simulink model "onelink_simscape"  (R2025a)
settings: Solver=ode15s  StartTime=0.0  StopTime=10  RelTol=1e-4
libraries: fl_lib x179, ee_lib x62, nesl_utility x15
(part 1 of 2)
settings Model: Creator=yang  LastModifiedBy=yang

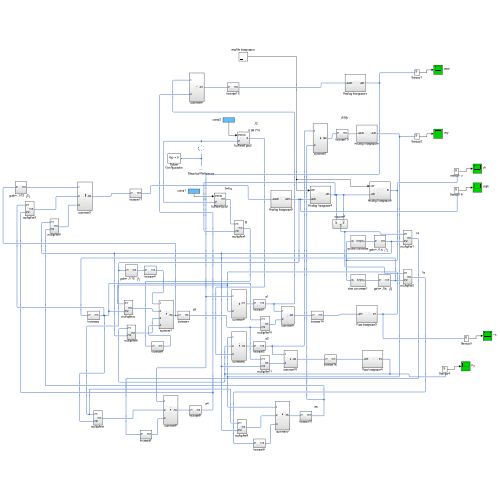
[thumbnail: Simulink's stored preview of the top-level diagram]
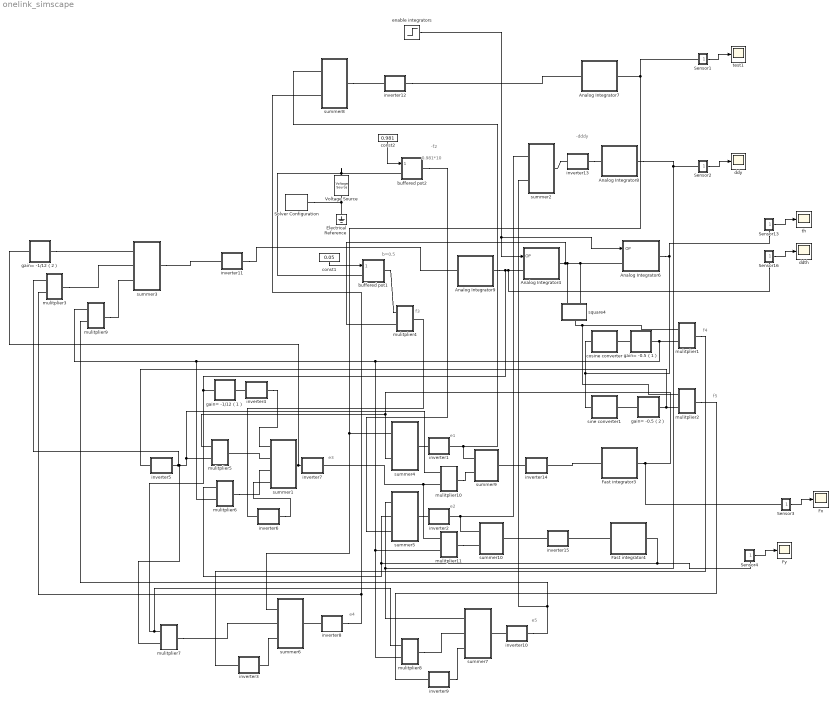
== system onelink_simscape ==
  note: 0.981*10
  note: -dddy
  note: e5
  note: e4
  note: e1
  note: f4
  note: f3
  note: b=0.5
  note: -f2
  note: f5
  note: e2
  note: e3
  Analog Integrator4 : Subsystem
  Analog Integrator6 : Subsystem
  Analog Integrator7 : Subsystem
  Analog Integrator8 : Subsystem
  Analog Integrator9 : Subsystem
  Electrical Reference : fl_lib/Electrical/Electrical Elements/Electrical Reference
  Fast integrator3 : Subsystem
  Fast integrator4 : Subsystem
  Fx : Scope
      settings: ActiveDisplayYMinimum=-37.571328229852568  ActiveDisplayYMaximum=27.796484303991519  DataLoggingVariableName=ScopeData4
  Fy : Scope
      settings: ActiveDisplayYMinimum=-21.350757214154832  ActiveDisplayYMaximum=2.3911956510501242  DataLoggingVariableName=ScopeData5
  Sensor1 : Subsystem
      mask Display: disp('S')
  Sensor13 : Subsystem
      settings: PortSchema="{\"entries\":[{\"content\":{\"sides\":[{\"content\":{},\"type\":\"ConnectorPlacement.EquallySpacedRectSide\",\"uuid\":\"8056b96b-3671-4774-a535-635e6b55e7ce\"},{\"content\":{\"connectorIds\":[\"Out1\"],\"side\":\"RIGHT\"},\"type\":\"ConnectorPlacement.EquallySpacedRectSide\",\"uuid\":\"d8cfde34-d3f1-4c6d-ab3a-246c7ad79664\"},{\"content\":{\"side\":\"TOP\"},\"type\":\"ConnectorPlacement.EquallySpacedRectSide\",\"uuid\":\"c78cfa8c-6b6c-49de-bc78-645cca7ac0e7\"},{\"content\":{\"connectorIds\":[\"RConn1\"],\"side\":\"BOTTOM\"},\"type\":\"ConnectorPlacement.EquallySpacedRectSide\",\"uuid\":\"959be980-bdc1-4803-beb2-1cc3f6e5a73d\"}]},\"type\":\"ConnectorPlacement.EquallySpacedConnector\",\"uuid\":\"4ae0772a-f601-42fd-b251-b1e340c12b80\"}],\"packageUris\":[\"http://schema.mathworks.com/mf0/Connector/R2020b\"],\"version\":\"1.0\"}"
      mask Display: disp('S')
  Sensor16 : Subsystem
      settings: PortSchema="{\"entries\":[{\"content\":{\"sides\":[{\"content\":{},\"type\":\"ConnectorPlacement.EquallySpacedRectSide\",\"uuid\":\"8056b96b-3671-4774-a535-635e6b55e7ce\"},{\"content\":{\"connectorIds\":[\"Out1\"],\"side\":\"RIGHT\"},\"type\":\"ConnectorPlacement.EquallySpacedRectSide\",\"uuid\":\"d8cfde34-d3f1-4c6d-ab3a-246c7ad79664\"},{\"content\":{\"side\":\"TOP\"},\"type\":\"ConnectorPlacement.EquallySpacedRectSide\",\"uuid\":\"c78cfa8c-6b6c-49de-bc78-645cca7ac0e7\"},{\"content\":{\"connectorIds\":[\"RConn1\"],\"side\":\"BOTTOM\"},\"type\":\"ConnectorPlacement.EquallySpacedRectSide\",\"uuid\":\"959be980-bdc1-4803-beb2-1cc3f6e5a73d\"}]},\"type\":\"ConnectorPlacement.EquallySpacedConnector\",\"uuid\":\"4ae0772a-f601-42fd-b251-b1e340c12b80\"}],\"packageUris\":[\"http://schema.mathworks.com/mf0/Connector/R2020b\"],\"version\":\"1.0\"}"
      mask Display: disp('S')
  Sensor2 : Subsystem
      mask Display: disp('S')
  Sensor3 : Subsystem
      mask Display: disp('S')
  Sensor4 : Subsystem
      settings: PortSchema="{\"entries\":[{\"content\":{\"sides\":[{\"content\":{},\"type\":\"ConnectorPlacement.EquallySpacedRectSide\",\"uuid\":\"8056b96b-3671-4774-a535-635e6b55e7ce\"},{\"content\":{\"connectorIds\":[\"Out1\"],\"side\":\"RIGHT\"},\"type\":\"ConnectorPlacement.EquallySpacedRectSide\",\"uuid\":\"d8cfde34-d3f1-4c6d-ab3a-246c7ad79664\"},{\"content\":{\"side\":\"TOP\"},\"type\":\"ConnectorPlacement.EquallySpacedRectSide\",\"uuid\":\"c78cfa8c-6b6c-49de-bc78-645cca7ac0e7\"},{\"content\":{\"connectorIds\":[\"RConn1\"],\"side\":\"BOTTOM\"},\"type\":\"ConnectorPlacement.EquallySpacedRectSide\",\"uuid\":\"959be980-bdc1-4803-beb2-1cc3f6e5a73d\"}]},\"type\":\"ConnectorPlacement.EquallySpacedConnector\",\"uuid\":\"4ae0772a-f601-42fd-b251-b1e340c12b80\"}],\"packageUris\":[\"http://schema.mathworks.com/mf0/Connector/R2020b\"],\"version\":\"1.0\"}"
      mask Display: disp('S')
  Solver Configuration : nesl_utility/Solver Configuration  PhysicalDomain=network_engine_domain  SubClassName=solver  LeftPortType=input  RightPortType=generic  Tones=[]  Harmonics=[]  SimulateNoise=off  Profile=off  UseLocalSampling=off  EnableSwitchedLinearOptims=on  FrequencyDomain=off  UseCCode=off  RelTol=0.001  AbsTol=1e-06  MinStep=1e-09  ToWorkspace=off  RevertToSquareIcSolve=off  NumHomotopyIterations=100  PhasorMode=off  PhasorModeNumHarmonics=1  ConsistencySolver=NEWTON_XTOL_AFTER_FTOL  IndexReductionMethod=DerivativeReplacement  DoDC=off  ResidualTolerance=1e-09  ConsistencyTolSource=GLOBAL  ConsistencyAbsTol=0.001  ConsistencyRelTol=0.001  ConsistencyTolFactor=0.001  UseLocalSolver=off  LocalSolverChoice=NE_BACKWARD_EULER_ADVANCER  ResolveIndetEquations=on  FunctionEvalNumThread=1  LocalSolverSampleTime=0.001  DoFixedCost=off  MaxNonlinIter=3  MaxModeIter=2  ComputeImpulses=off  ImpulseIterations=2  LinearAlgebra=auto  LinearAlgebraNumThread=0  EquationFormulation=NE_TIME_EF  DelaysMemoryBudget=1024  AutomaticFiltering=on  FilteringTimeConstant=0.001  PartitionStorageMethod=AS_NEEDED  PartitionMemoryBudget=1024  PartitionMethod=ROBUST  MultibodyUseLocalSolver=off  MultibodyLocalSolverChoice=ODE1  MultibodyLocalSolverSampleTime=0.001
  Voltage Source : ee_lib/Sources/Voltage Source  dc_voltage=10 V  ac_voltage=0 V  ac_shift=0 rad  ac_frequency=60 Hz  noise_mode=ee.enum.sources.noise.Disabled  PSD=0 V^2/Hz  sample_time=1e-3 s  repeatability=ee.enum.sources.repeatability.NotRepeatable  user_seed=0  auto_seed=3499211588  i_specify=off  i_priority=None  i=0 A  i_nominal_specify=off  i_nominal_value=1  i_nominal_unit=A  v_specify=off  v_priority=None  v=0 V  v_nominal_specify=off  v_nominal_value=1  v_nominal_unit=V
  buffered pot1 : Subsystem
  buffered pot2 : Subsystem
  const1 : Constant  Value=0.05
  const2 : Constant  Value=0.981
  cosine converter : Subsystem
  ddth : Scope
      settings: ActiveDisplayYMinimum=-17.651400313660709  ActiveDisplayYMaximum=14.639431018318287
  ddy : Scope
      settings: ActiveDisplayYMinimum=-8.0449324202485482  ActiveDisplayYMaximum=0.91267312902724274  DataLoggingVariableName=ScopeData3
  enable integrators : Step  Time=0.02  SampleTime=0
  gain= -0.5（1） : Subsystem
  gain= -0.5（2） : Subsystem
  gain= -1/12（1） : Subsystem
  gain= -1/12（2） : Subsystem
  inverter1 : Subsystem
  inverter10 : Subsystem
  inverter11 : Subsystem
  inverter12 : Subsystem
  inverter13 : Subsystem
  inverter14 : Subsystem
  inverter15 : Subsystem
  inverter2 : Subsystem
  inverter3 : Subsystem
  inverter4 : Subsystem
  inverter5 : Subsystem
  inverter6 : Subsystem
  inverter7 : Subsystem
  inverter8 : Subsystem
  inverter9 : Subsystem
  mulitplier1 : Subsystem
  mulitplier10 : Subsystem
  mulitplier11 : Subsystem
  mulitplier2 : Subsystem
  mulitplier3 : Subsystem
  mulitplier4 : Subsystem
  mulitplier5 : Subsystem
  mulitplier6 : Subsystem
  mulitplier7 : Subsystem
  mulitplier8 : Subsystem
  mulitplier9 : Subsystem
  sine converter1 : Subsystem
  square4 : Subsystem
  summer1 : Subsystem
  summer10 : Subsystem
  summer2 : Subsystem
  summer3 : Subsystem
  summer4 : Subsystem
  summer5 : Subsystem
  summer6 : Subsystem
  summer7 : Subsystem
  summer8 : Subsystem
  summer9 : Subsystem
  test1 : Scope
      settings: ActiveDisplayYMinimum=-5.82803  ActiveDisplayYMaximum=0.09194
  th : Scope
      settings: ActiveDisplayYMinimum=-2.64598748843829  ActiveDisplayYMaximum=0.29399860983456916  DataLoggingVariableName=ScopeData14
  wires:
  const2/1 -> buffered pot2/1(input0)
  enable integrators/1 -> Analog Integrator6/1(OP), Analog Integrator4/1(OP)
  const1/1 -> buffered pot1/1(input0)
  Sensor16/1(Out1) -> ddth/1
  Sensor1/1(Out1) -> test1/1
  Sensor2/1(Out1) -> ddy/1
  Sensor3/1(Out1) -> Fx/1
  Sensor4/1(Out1) -> Fy/1
  Sensor13/1(Out1) -> th/1
  connections:
  Solver Configuration/RConn1 -- Voltage Source/RConn1 -- Electrical Reference/LConn1
  Voltage Source/LConn1 -- buffered pot1/LConn1 -- buffered pot2/LConn1
  Analog Integrator4/RConn1 -- mulitplier4/LConn2 -- square4/LConn1 -- square4/LConn2 -- Analog Integrator6/LConn1
  buffered pot1/RConn1 -- mulitplier4/LConn1
  mulitplier1/LConn1 -- mulitplier2/LConn1 -- square4/RConn1
  Analog Integrator6/RConn1 -- sine converter1/LConn1 -- cosine converter/LConn1 -- Sensor13/RConn1
  Analog Integrator9/RConn1 -- Sensor16/RConn1 -- Analog Integrator4/LConn1 -- mulitplier8/LConn1 -- mulitplier7/LConn1 -- gain= -1/12（1）/LConn1
  summer4/LConn1 -- summer6/LConn1 -- Sensor1/LConn1 -- Analog Integrator7/RConn1
  Fast integrator3/RConn1 -- Sensor3/LConn1 -- mulitplier5/LConn1 -- summer4/LConn2
  inverter1/LConn1 -- summer4/RConn1
  Analog Integrator8/RConn1 -- Sensor2/LConn1 -- summer7/LConn1 -- summer5/LConn1
  summer5/LConn2 -- mulitplier6/LConn1 -- Sensor4/RConn1 -- Fast integrator4/RConn1
  buffered pot2/RConn1 -- summer5/LConn3
  inverter2/LConn1 -- summer5/RConn1
  inverter4/LConn1 -- gain= -1/12（1）/RConn1
  inverter4/RConn1 -- summer1/LConn1
  gain= -0.5（1）/LConn1 -- cosine converter/RConn1
  mulitplier1/LConn2 -- mulitplier11/LConn2 -- mulitplier8/LConn2 -- mulitplier9/LConn1 -- mulitplier6/LConn2 -- gain= -0.5（1）/RConn1
  gain= -0.5（2）/LConn1 -- sine converter1/RConn1
  mulitplier2/LConn2 -- inverter5/LConn1 -- gain= -0.5（2）/RConn1
  inverter5/RConn1 -- mulitplier3/LConn1 -- mulitplier7/LConn2 -- mulitplier10/LConn1 -- mulitplier5/LConn2
  summer1/LConn2 -- mulitplier5/RConn1
  mulitplier6/RConn1 -- summer1/LConn3
  inverter6/LConn1 -- mulitplier4/RConn1
  inverter6/RConn1 -- summer1/LConn4
  inverter7/LConn1 -- gain= -1/12（2）/LConn1 -- summer1/RConn1
  mulitplier7/RConn1 -- summer6/LConn2
  mulitplier1/RConn1 -- inverter3/LConn1
  summer6/LConn3 -- inverter3/RConn1
  inverter8/LConn1 -- summer6/RConn1
  mulitplier8/RConn1 -- summer7/LConn2
  mulitplier2/RConn1 -- inverter9/LConn1
  inverter9/RConn1 -- summer7/LConn3
  inverter10/LConn1 -- summer7/RConn1
  summer8/LConn1 -- summer9/LConn1 -- inverter1/RConn1
  inverter8/RConn1 -- mulitplier3/LConn2 -- summer8/LConn2
  summer8/RConn1 -- inverter12/LConn1
  inverter12/RConn1 -- Analog Integrator7/LConn1
  summer2/LConn1 -- summer10/LConn1 -- inverter2/RConn1
  inverter10/RConn1 -- mulitplier9/LConn2 -- summer2/LConn2
  inverter13/LConn1 -- summer2/RConn1
  inverter13/RConn1 -- Analog Integrator8/LConn1
  gain= -1/12（2）/RConn1 -- summer3/LConn1
  mulitplier3/RConn1 -- summer3/LConn2
  mulitplier9/RConn1 -- summer3/LConn3
  mulitplier10/LConn2 -- inverter7/RConn1 -- mulitplier11/LConn1
  mulitplier10/RConn1 -- summer9/LConn2
  inverter14/LConn1 -- summer9/RConn1
  Fast integrator3/LConn1 -- inverter14/RConn1
  inverter15/LConn1 -- summer10/RConn1
  Fast integrator4/LConn1 -- inverter15/RConn1
  mulitplier11/RConn1 -- summer10/LConn2
  summer3/RConn1 -- inverter11/LConn1
  inverter11/RConn1 -- Analog Integrator9/LConn1

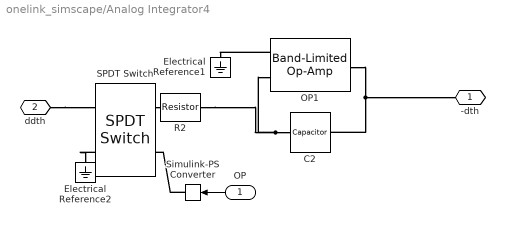
== system onelink_simscape/Analog Integrator4 ==
  OP : Inport
  C2 : ee_lib/Passive/Capacitor  cap_option=ee.enum.passive.capacitor.capOption.const  c=1e-6 F  Cvec=[1e-05, 1e-06] F  Vvec=[0, 10] V  CV_table_symmetry=ee.enum.passive.capacitor.tableSymmetry.yes  f_vec=[1, 10] kHz  DFext_vec=[.8, 1.2]  enable_C_tol=ee.enum.toleranceApplication.none  averaging_period=0 s  C_tol=5  tol_distribution=ee.enum.toleranceDistribution.uniform  nSigma=4  r=1e-6 Ohm  g=0 1/Ohm  enable_operating_limits=ee.enum.enable.no  operating_limit_action=ee.enum.passive.reportOpLim.warn  max_working_voltage_range=[-25, 25] V  power_rating=1 W  maxTemperature=85 degC  thermalEnable=false  thermalMass=1 J/K  i_specify=off  i_priority=None  i=0 A  i_nominal_specify=off  i_nominal_value=1  i_nominal_unit=A  v_specify=off  v_priority=High  v=1 V  v_nominal_specify=off  v_nominal_value=1  v_nominal_unit=V  vc_specify=on  vc_priority=High  vc=0 V  vc_nominal_specify=off  vc_nominal_value=1  vc_nominal_unit=V  T_specify=off  T_priority=None  T=298.15 K  T_nominal_specify=off  T_nominal_value=1  T_nominal_unit=K
  Electrical Reference1 : fl_lib/Electrical/Electrical Elements/Electrical Reference
  Electrical Reference2 : fl_lib/Electrical/Electrical Elements/Electrical Reference
  OP1 : ee_lib/Integrated Circuits/Band-Limited Op-Amp  A=1.8E6  Rin=1 GOhm  Rout=70 Ohm  Vmin=-15 V  Vmax=15 V  Vdotmax=2.8E6 V/s  f=8E6 Hz  V0=0 V
  R2 : fl_lib/Electrical/Electrical Elements/Resistor  R=1E6 Ohm  i_specify=off  i_priority=None  i=0 A  i_nominal_specify=off  i_nominal_value=1  i_nominal_unit=A  v_specify=off  v_priority=None  v=0 V  v_nominal_specify=off  v_nominal_value=1  v_nominal_unit=V
  SPDT Switch : ee_lib/Switches & Breakers/SPDT Switch  R_closed=0.01 Ohm  G_open=1e-6 S  Threshold=0.5 V  Width=0 V  model_dynamics=0  t_on=1e-3 s  t_off=1e-3 s  initial_vT=0 V
  Simulink-PS Converter : nesl_utility/Simulink-PS Converter  PhysicalDomain=network_engine_domain  SubClassName=ps_input  LeftPortType=input  RightPortType=output  PseudoPeriodic=off  Frequencies=[]  NoiseDistribution=none  NoiseParameters=[]  Unit=1  AffineConversion=off  FilteringAndDerivatives=provide  SimscapeFilterOrder=1  InputFilterTimeConstant=0.001  UdotUserProvided=0
  -dth : PMIOPort  Side=Right
  ddth : PMIOPort  Port=2  Side=Left
  wires:
  OP/1 -> Simulink-PS Converter/1
  connections:
  Simulink-PS Converter/RConn1 -- SPDT Switch/LConn1
  SPDT Switch/RConn1 -- Electrical Reference2/LConn1
  ddth/RConn1 -- SPDT Switch/RConn2
  SPDT Switch/LConn2 -- R2/LConn1
  OP1/RConn1 -- -dth/RConn1 -- C2/RConn1
  C2/LConn1 -- OP1/LConn2 -- R2/RConn1
  OP1/LConn1 -- Electrical Reference1/LConn1

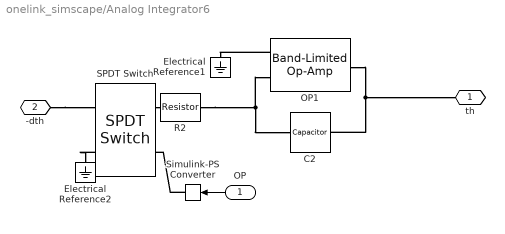
== system onelink_simscape/Analog Integrator6 ==
  OP : Inport
  C2 : ee_lib/Passive/Capacitor  cap_option=ee.enum.passive.capacitor.capOption.const  c=1e-6 F  Cvec=[1e-05, 1e-06] F  Vvec=[0, 10] V  CV_table_symmetry=ee.enum.passive.capacitor.tableSymmetry.yes  f_vec=[1, 10] kHz  DFext_vec=[.8, 1.2]  enable_C_tol=ee.enum.toleranceApplication.none  averaging_period=0 s  C_tol=5  tol_distribution=ee.enum.toleranceDistribution.uniform  nSigma=4  r=1e-6 Ohm  g=0 1/Ohm  enable_operating_limits=ee.enum.enable.no  operating_limit_action=ee.enum.passive.reportOpLim.warn  max_working_voltage_range=[-25, 25] V  power_rating=1 W  maxTemperature=85 degC  thermalEnable=false  thermalMass=1 J/K  i_specify=off  i_priority=None  i=0 A  i_nominal_specify=off  i_nominal_value=1  i_nominal_unit=A  v_specify=off  v_priority=High  v=1 V  v_nominal_specify=off  v_nominal_value=1  v_nominal_unit=V  vc_specify=on  vc_priority=High  vc=0 V  vc_nominal_specify=off  vc_nominal_value=1  vc_nominal_unit=V  T_specify=off  T_priority=None  T=298.15 K  T_nominal_specify=off  T_nominal_value=1  T_nominal_unit=K
  Electrical Reference1 : fl_lib/Electrical/Electrical Elements/Electrical Reference
  Electrical Reference2 : fl_lib/Electrical/Electrical Elements/Electrical Reference
  OP1 : ee_lib/Integrated Circuits/Band-Limited Op-Amp  A=1.8E6  Rin=1 GOhm  Rout=70 Ohm  Vmin=-15 V  Vmax=15 V  Vdotmax=2.8E6 V/s  f=8E6 Hz  V0=0 V
  R2 : fl_lib/Electrical/Electrical Elements/Resistor  R=1E6 Ohm  i_specify=off  i_priority=None  i=0 A  i_nominal_specify=off  i_nominal_value=1  i_nominal_unit=A  v_specify=off  v_priority=None  v=0 V  v_nominal_specify=off  v_nominal_value=1  v_nominal_unit=V
  SPDT Switch : ee_lib/Switches & Breakers/SPDT Switch  R_closed=0.01 Ohm  G_open=1e-6 S  Threshold=0.5 V  Width=0 V  model_dynamics=0  t_on=1e-3 s  t_off=1e-3 s  initial_vT=0 V
  Simulink-PS Converter : nesl_utility/Simulink-PS Converter  PhysicalDomain=network_engine_domain  SubClassName=ps_input  LeftPortType=input  RightPortType=output  PseudoPeriodic=off  Frequencies=[]  NoiseDistribution=none  NoiseParameters=[]  Unit=1  AffineConversion=off  FilteringAndDerivatives=provide  SimscapeFilterOrder=1  InputFilterTimeConstant=0.001  UdotUserProvided=0
  th : PMIOPort  Side=Right
  -dth : PMIOPort  Port=2  Side=Left
  wires:
  OP/1 -> Simulink-PS Converter/1
  connections:
  OP1/LConn1 -- Electrical Reference1/LConn1
  R2/RConn1 -- OP1/LConn2 -- C2/LConn1
  C2/RConn1 -- th/RConn1 -- OP1/RConn1
  SPDT Switch/LConn2 -- R2/LConn1
  -dth/RConn1 -- SPDT Switch/RConn2
  SPDT Switch/RConn1 -- Electrical Reference2/LConn1
  Simulink-PS Converter/RConn1 -- SPDT Switch/LConn1

== system onelink_simscape/Analog Integrator7 ==
  C2 : ee_lib/Passive/Capacitor  cap_option=ee.enum.passive.capacitor.capOption.const  c=10 nF  Cvec=[1e-05, 1e-06] F  Vvec=[0, 10] V  CV_table_symmetry=ee.enum.passive.capacitor.tableSymmetry.yes  f_vec=[1, 10] kHz  DFext_vec=[.8, 1.2]  enable_C_tol=ee.enum.toleranceApplication.none  averaging_period=0 s  C_tol=5  tol_distribution=ee.enum.toleranceDistribution.uniform  nSigma=4  r=1e-6 Ohm  g=0 1/Ohm  enable_operating_limits=ee.enum.enable.no  operating_limit_action=ee.enum.passive.reportOpLim.warn  max_working_voltage_range=[-25, 25] V  power_rating=1 W  maxTemperature=85 degC  thermalEnable=false  thermalMass=1 J/K  i_specify=off  i_priority=None  i=0 A  i_nominal_specify=off  i_nominal_value=1  i_nominal_unit=A  v_specify=off  v_priority=High  v=1 V  v_nominal_specify=off  v_nominal_value=1  v_nominal_unit=V  vc_specify=on  vc_priority=High  vc=0 V  vc_nominal_specify=off  vc_nominal_value=1  vc_nominal_unit=V  T_specify=off  T_priority=None  T=298.15 K  T_nominal_specify=off  T_nominal_value=1  T_nominal_unit=K
  Electrical Reference1 : fl_lib/Electrical/Electrical Elements/Electrical Reference
  OP1 : ee_lib/Integrated Circuits/Band-Limited Op-Amp  A=1.8E6  Rin=4e6 Ohm  Rout=70 Ohm  Vmin=-15 V  Vmax=15 V  Vdotmax=2.8E6 V/s  f=8E6 Hz  V0=0 V
  R2 : fl_lib/Electrical/Electrical Elements/Resistor  R=33.3 kOhm  i_specify=off  i_priority=None  i=0 A  i_nominal_specify=off  i_nominal_value=1  i_nominal_unit=A  v_specify=off  v_priority=None  v=0 V  v_nominal_specify=off  v_nominal_value=1  v_nominal_unit=V
  ddx : PMIOPort  Side=Right
  -dddx : PMIOPort  Port=2  Side=Left
  connections:
  OP1/LConn1 -- Electrical Reference1/LConn1
  R2/RConn1 -- OP1/LConn2 -- C2/LConn1
  C2/RConn1 -- ddx/RConn1 -- OP1/RConn1
  -dddx/RConn1 -- R2/LConn1

== system onelink_simscape/Analog Integrator8 ==
  C2 : ee_lib/Passive/Capacitor  cap_option=ee.enum.passive.capacitor.capOption.const  c=10 nF  Cvec=[1e-05, 1e-06] F  Vvec=[0, 10] V  CV_table_symmetry=ee.enum.passive.capacitor.tableSymmetry.yes  f_vec=[1, 10] kHz  DFext_vec=[.8, 1.2]  enable_C_tol=ee.enum.toleranceApplication.none  averaging_period=0 s  C_tol=5  tol_distribution=ee.enum.toleranceDistribution.uniform  nSigma=4  r=1e-6 Ohm  g=0 1/Ohm  enable_operating_limits=ee.enum.enable.no  operating_limit_action=ee.enum.passive.reportOpLim.warn  max_working_voltage_range=[-25, 25] V  power_rating=1 W  maxTemperature=85 degC  thermalEnable=false  thermalMass=1 J/K  i_specify=off  i_priority=None  i=0 A  i_nominal_specify=off  i_nominal_value=1  i_nominal_unit=A  v_specify=off  v_priority=High  v=1 V  v_nominal_specify=off  v_nominal_value=1  v_nominal_unit=V  vc_specify=on  vc_priority=High  vc=0 V  vc_nominal_specify=off  vc_nominal_value=1  vc_nominal_unit=V  T_specify=off  T_priority=None  T=298.15 K  T_nominal_specify=off  T_nominal_value=1  T_nominal_unit=K
  Electrical Reference1 : fl_lib/Electrical/Electrical Elements/Electrical Reference
  OP1 : ee_lib/Integrated Circuits/Band-Limited Op-Amp  A=1.8E6  Rin=4e6 Ohm  Rout=70 Ohm  Vmin=-15 V  Vmax=15 V  Vdotmax=2.8E6 V/s  f=8E6 Hz  V0=0 V
  R2 : fl_lib/Electrical/Electrical Elements/Resistor  R=33.3 kOhm  i_specify=off  i_priority=None  i=0 A  i_nominal_specify=off  i_nominal_value=1  i_nominal_unit=A  v_specify=off  v_priority=None  v=0 V  v_nominal_specify=off  v_nominal_value=1  v_nominal_unit=V
  ddy : PMIOPort  Side=Right
  -dddy : PMIOPort  Port=2  Side=Left
  connections:
  -dddy/RConn1 -- R2/LConn1
  OP1/RConn1 -- ddy/RConn1 -- C2/RConn1
  C2/LConn1 -- OP1/LConn2 -- R2/RConn1
  OP1/LConn1 -- Electrical Reference1/LConn1

== system onelink_simscape/Analog Integrator9 ==
  C2 : ee_lib/Passive/Capacitor  cap_option=ee.enum.passive.capacitor.capOption.const  c=10 nF  Cvec=[1e-05, 1e-06] F  Vvec=[0, 10] V  CV_table_symmetry=ee.enum.passive.capacitor.tableSymmetry.yes  f_vec=[1, 10] kHz  DFext_vec=[.8, 1.2]  enable_C_tol=ee.enum.toleranceApplication.none  averaging_period=0 s  C_tol=5  tol_distribution=ee.enum.toleranceDistribution.uniform  nSigma=4  r=1e-6 Ohm  g=0 1/Ohm  enable_operating_limits=ee.enum.enable.no  operating_limit_action=ee.enum.passive.reportOpLim.warn  max_working_voltage_range=[-25, 25] V  power_rating=1 W  maxTemperature=85 degC  thermalEnable=false  thermalMass=1 J/K  i_specify=off  i_priority=None  i=0 A  i_nominal_specify=off  i_nominal_value=1  i_nominal_unit=A  v_specify=off  v_priority=High  v=1 V  v_nominal_specify=off  v_nominal_value=1  v_nominal_unit=V  vc_specify=on  vc_priority=High  vc=0 V  vc_nominal_specify=off  vc_nominal_value=1  vc_nominal_unit=V  T_specify=off  T_priority=None  T=298.15 K  T_nominal_specify=off  T_nominal_value=1  T_nominal_unit=K
  Electrical Reference1 : fl_lib/Electrical/Electrical Elements/Electrical Reference
  OP1 : ee_lib/Integrated Circuits/Band-Limited Op-Amp  A=1.8E6  Rin=4e6 GOhm  Rout=70 Ohm  Vmin=-24 V  Vmax=24 V  Vdotmax=2.8E6 V/s  f=8E6 Hz  V0=0 V
  R1 : fl_lib/Electrical/Electrical Elements/Resistor  R=50 MOhm  i_specify=off  i_priority=None  i=0 A  i_nominal_specify=off  i_nominal_value=1  i_nominal_unit=A  v_specify=off  v_priority=None  v=0 V  v_nominal_specify=off  v_nominal_value=1  v_nominal_unit=V
  R2 : fl_lib/Electrical/Electrical Elements/Resistor  R=33.3 kOhm  i_specify=off  i_priority=None  i=0 A  i_nominal_specify=off  i_nominal_value=1  i_nominal_unit=A  v_specify=off  v_priority=None  v=0 V  v_nominal_specify=off  v_nominal_value=1  v_nominal_unit=V
  ddth : PMIOPort  Side=Right
  -dddth : PMIOPort  Port=2  Side=Left
  connections:
  OP1/LConn1 -- Electrical Reference1/LConn1
  R2/RConn1 -- OP1/LConn2 -- R1/LConn1 -- C2/LConn1
  OP1/RConn1 -- ddth/RConn1 -- R1/RConn1 -- C2/RConn1
  -dddth/RConn1 -- R2/LConn1

== system onelink_simscape/Fast integrator3 ==
  C2 : ee_lib/Passive/Capacitor  cap_option=ee.enum.passive.capacitor.capOption.const  c=10 nF  Cvec=[1e-05, 1e-06] F  Vvec=[0, 10] V  CV_table_symmetry=ee.enum.passive.capacitor.tableSymmetry.yes  f_vec=[1, 10] kHz  DFext_vec=[.8, 1.2]  enable_C_tol=ee.enum.toleranceApplication.none  averaging_period=0 s  C_tol=5  tol_distribution=ee.enum.toleranceDistribution.uniform  nSigma=4  r=1e-6 Ohm  g=0 1/Ohm  enable_operating_limits=ee.enum.enable.no  operating_limit_action=ee.enum.passive.reportOpLim.warn  max_working_voltage_range=[-25, 25] V  power_rating=1 W  maxTemperature=85 degC  thermalEnable=false  thermalMass=1 J/K  i_specify=off  i_priority=None  i=0 A  i_nominal_specify=off  i_nominal_value=1  i_nominal_unit=A  v_specify=off  v_priority=High  v=1 V  v_nominal_specify=off  v_nominal_value=1  v_nominal_unit=V  vc_specify=on  vc_priority=High  vc=0 V  vc_nominal_specify=off  vc_nominal_value=1  vc_nominal_unit=V  T_specify=off  T_priority=None  T=298.15 K  T_nominal_specify=off  T_nominal_value=1  T_nominal_unit=K
  Electrical Reference1 : fl_lib/Electrical/Electrical Elements/Electrical Reference
  OP1 : ee_lib/Integrated Circuits/Band-Limited Op-Amp  A=1.8E6  Rin=4e6 Ohm  Rout=70 Ohm  Vmin=-24 V  Vmax=24 V  Vdotmax=2.8E6 V/s  f=8E6 Hz  V0=0 V
  R2 : fl_lib/Electrical/Electrical Elements/Resistor  R=33.3 kOhm  i_specify=off  i_priority=None  i=0 A  i_nominal_specify=off  i_nominal_value=1  i_nominal_unit=A  v_specify=off  v_priority=None  v=0 V  v_nominal_specify=off  v_nominal_value=1  v_nominal_unit=V
  Fx : PMIOPort  Side=Right
  -dFx : PMIOPort  Port=2  Side=Left
  connections:
  OP1/RConn1 -- C2/RConn1 -- Fx/RConn1
  C2/LConn1 -- R2/RConn1 -- OP1/LConn2
  OP1/LConn1 -- Electrical Reference1/LConn1
  R2/LConn1 -- -dFx/RConn1

== system onelink_simscape/Fast integrator4 ==
  C2 : ee_lib/Passive/Capacitor  cap_option=ee.enum.passive.capacitor.capOption.const  c=10 nF  Cvec=[1e-05, 1e-06] F  Vvec=[0, 10] V  CV_table_symmetry=ee.enum.passive.capacitor.tableSymmetry.yes  f_vec=[1, 10] kHz  DFext_vec=[.8, 1.2]  enable_C_tol=ee.enum.toleranceApplication.none  averaging_period=0 s  C_tol=5  tol_distribution=ee.enum.toleranceDistribution.uniform  nSigma=4  r=1e-6 Ohm  g=0 1/Ohm  enable_operating_limits=ee.enum.enable.no  operating_limit_action=ee.enum.passive.reportOpLim.warn  max_working_voltage_range=[-25, 25] V  power_rating=1 W  maxTemperature=85 degC  thermalEnable=false  thermalMass=1 J/K  i_specify=off  i_priority=None  i=0 A  i_nominal_specify=off  i_nominal_value=1  i_nominal_unit=A  v_specify=off  v_priority=High  v=1 V  v_nominal_specify=off  v_nominal_value=1  v_nominal_unit=V  vc_specify=on  vc_priority=High  vc=0 V  vc_nominal_specify=off  vc_nominal_value=1  vc_nominal_unit=V  T_specify=off  T_priority=None  T=298.15 K  T_nominal_specify=off  T_nominal_value=1  T_nominal_unit=K
  Electrical Reference1 : fl_lib/Electrical/Electrical Elements/Electrical Reference
  OP1 : ee_lib/Integrated Circuits/Band-Limited Op-Amp  A=1.8E6  Rin=4e6 Ohm  Rout=70 Ohm  Vmin=-24 V  Vmax=24 V  Vdotmax=28E6 V/s  f=8E6 Hz  V0=0 V
  R2 : fl_lib/Electrical/Electrical Elements/Resistor  R=33.3 kOhm  i_specify=off  i_priority=None  i=0 A  i_nominal_specify=off  i_nominal_value=1  i_nominal_unit=A  v_specify=off  v_priority=None  v=0 V  v_nominal_specify=off  v_nominal_value=1  v_nominal_unit=V
  Fy : PMIOPort  Side=Right
  -dFy : PMIOPort  Port=2  Side=Left
  connections:
  OP1/LConn1 -- Electrical Reference1/LConn1
  R2/RConn1 -- OP1/LConn2 -- C2/LConn1
  Fy/RConn1 -- C2/RConn1 -- OP1/RConn1
  -dFy/RConn1 -- R2/LConn1

== system onelink_simscape/Sensor1 ==
  ERef : fl_lib/Electrical/Electrical Elements/Electrical Reference
  PS-Simulink Converter : nesl_utility/PS-Simulink Converter  PhysicalDomain=network_engine_domain  SubClassName=ps_output  LeftPortType=input  RightPortType=output  PseudoPeriodic=off  Frequencies=[]  VectorFormat=1-D array  Unit=1  AffineConversion=off
  Voltage Sensor : fl_lib/Electrical/Electrical Sensors/Voltage Sensor
  Conn1 : PMIOPort  Side=Left
  Out1 : Outport  VectorParamsAs1DForOutWhenUnconnected=off
  wires:
  PS-Simulink Converter/1 -> Out1/1
  connections:
  ERef/LConn1 -- Voltage Sensor/RConn2
  Voltage Sensor/RConn1 -- PS-Simulink Converter/LConn1
  Voltage Sensor/LConn1 -- Conn1/RConn1

== system onelink_simscape/Sensor13 ==
  ERef : fl_lib/Electrical/Electrical Elements/Electrical Reference
  PS-Simulink Converter : nesl_utility/PS-Simulink Converter  PhysicalDomain=network_engine_domain  SubClassName=ps_output  LeftPortType=input  RightPortType=output  PseudoPeriodic=off  Frequencies=[]  VectorFormat=1-D array  Unit=1  AffineConversion=off
  Voltage Sensor : fl_lib/Electrical/Electrical Sensors/Voltage Sensor
  Conn1 : PMIOPort  Side=Right
  Out1 : Outport  VectorParamsAs1DForOutWhenUnconnected=off
  wires:
  PS-Simulink Converter/1 -> Out1/1
  connections:
  ERef/LConn1 -- Voltage Sensor/RConn2
  Voltage Sensor/RConn1 -- PS-Simulink Converter/LConn1
  Voltage Sensor/LConn1 -- Conn1/RConn1

== system onelink_simscape/Sensor16 ==
  ERef : fl_lib/Electrical/Electrical Elements/Electrical Reference
  PS-Simulink Converter : nesl_utility/PS-Simulink Converter  PhysicalDomain=network_engine_domain  SubClassName=ps_output  LeftPortType=input  RightPortType=output  PseudoPeriodic=off  Frequencies=[]  VectorFormat=1-D array  Unit=1  AffineConversion=off
  Voltage Sensor : fl_lib/Electrical/Electrical Sensors/Voltage Sensor
  Conn1 : PMIOPort  Side=Right
  Out1 : Outport  VectorParamsAs1DForOutWhenUnconnected=off
  wires:
  PS-Simulink Converter/1 -> Out1/1
  connections:
  ERef/LConn1 -- Voltage Sensor/RConn2
  Voltage Sensor/RConn1 -- PS-Simulink Converter/LConn1
  Voltage Sensor/LConn1 -- Conn1/RConn1

== system onelink_simscape/Sensor2 ==
  ERef : fl_lib/Electrical/Electrical Elements/Electrical Reference
  PS-Simulink Converter : nesl_utility/PS-Simulink Converter  PhysicalDomain=network_engine_domain  SubClassName=ps_output  LeftPortType=input  RightPortType=output  PseudoPeriodic=off  Frequencies=[]  VectorFormat=1-D array  Unit=1  AffineConversion=off
  Voltage Sensor : fl_lib/Electrical/Electrical Sensors/Voltage Sensor
  Conn1 : PMIOPort  Side=Left
  Out1 : Outport  VectorParamsAs1DForOutWhenUnconnected=off
  wires:
  PS-Simulink Converter/1 -> Out1/1
  connections:
  ERef/LConn1 -- Voltage Sensor/RConn2
  Voltage Sensor/RConn1 -- PS-Simulink Converter/LConn1
  Voltage Sensor/LConn1 -- Conn1/RConn1

== system onelink_simscape/Sensor3 ==
  ERef : fl_lib/Electrical/Electrical Elements/Electrical Reference
  PS-Simulink Converter : nesl_utility/PS-Simulink Converter  PhysicalDomain=network_engine_domain  SubClassName=ps_output  LeftPortType=input  RightPortType=output  PseudoPeriodic=off  Frequencies=[]  VectorFormat=1-D array  Unit=1  AffineConversion=off
  Voltage Sensor : fl_lib/Electrical/Electrical Sensors/Voltage Sensor
  Conn1 : PMIOPort  Side=Left
  Out1 : Outport  VectorParamsAs1DForOutWhenUnconnected=off
  wires:
  PS-Simulink Converter/1 -> Out1/1
  connections:
  ERef/LConn1 -- Voltage Sensor/RConn2
  Voltage Sensor/RConn1 -- PS-Simulink Converter/LConn1
  Voltage Sensor/LConn1 -- Conn1/RConn1

== system onelink_simscape/Sensor4 ==
  ERef : fl_lib/Electrical/Electrical Elements/Electrical Reference
  PS-Simulink Converter : nesl_utility/PS-Simulink Converter  PhysicalDomain=network_engine_domain  SubClassName=ps_output  LeftPortType=input  RightPortType=output  PseudoPeriodic=off  Frequencies=[]  VectorFormat=1-D array  Unit=1  AffineConversion=off
  Voltage Sensor : fl_lib/Electrical/Electrical Sensors/Voltage Sensor
  Conn1 : PMIOPort  Side=Right
  Out1 : Outport  VectorParamsAs1DForOutWhenUnconnected=off
  wires:
  PS-Simulink Converter/1 -> Out1/1
  connections:
  ERef/LConn1 -- Voltage Sensor/RConn2
  Voltage Sensor/RConn1 -- PS-Simulink Converter/LConn1
  Voltage Sensor/LConn1 -- Conn1/RConn1

== system onelink_simscape/buffered pot1 ==
  input0 : Inport
  Electrical Reference4 : fl_lib/Electrical/Electrical Elements/Electrical Reference
  OP4 : ee_lib/Integrated Circuits/Band-Limited Op-Amp  A=1.8E6  Rin=4e6 Ohm  Rout=70 Ohm  Vmin=-24 V  Vmax=24 V  Vdotmax=2.8E6 V/s  f=8E6 Hz  V0=0 V
  Potentiometer : ee_lib/Passive/Potentiometer  nPorts=ee.enum.passive.potentiometer.nPorts.Three  R0=10E3 Ohm  Rw=1 Ohm  xmin=0  xmax=1  minResistance=1 Ohm  maxResistance=999 Ohm  xmin2port=0  xmax2port=1  Taper=ee.enum.passive.potentiometer.linOrLog.lin  Rcenter=200 Ohm  Gradient=ee.enum.passive.potentiometer.gradient.higherR
      settings: InternalSimscapePortConfiguration="{\"Bottom\":[],\"Left\":[{\"id\":\"pinL\",\"label\":\"L\",\"type\":\"foundation.electrical.electrical\"},{\"id\":\"W\",\"label\":\"W\",\"type\":\"foundation.electrical.electrical\"}],\"Right\":[{\"id\":\"pinR\",\"label\":\"R\",\"type\":\"foundation.electrical.electrical\"},{\"id\":\"x\",\"label\":\"x\",\"type\":\"input\"}],\"Top\":[]}"
  Simulink-PS Converter : nesl_utility/Simulink-PS Converter  PhysicalDomain=network_engine_domain  SubClassName=ps_input  LeftPortType=input  RightPortType=output  PseudoPeriodic=off  Frequencies=[]  NoiseDistribution=none  NoiseParameters=[]  Unit=1  AffineConversion=off  FilteringAndDerivatives=provide  SimscapeFilterOrder=1  InputFilterTimeConstant=0.001  UdotUserProvided=0
  out : PMIOPort  Side=Right
  in : PMIOPort  Port=2  Side=Left
  wires:
  input0/1 -> Simulink-PS Converter/1
  connections:
  in/RConn1 -- Potentiometer/RConn1
  OP4/LConn2 -- out/RConn1 -- OP4/RConn1
  Electrical Reference4/LConn1 -- Potentiometer/LConn1
  Potentiometer/LConn2 -- OP4/LConn1
  Simulink-PS Converter/RConn1 -- Potentiometer/RConn2

== system onelink_simscape/buffered pot2 ==
  input0 : Inport
  Electrical Reference4 : fl_lib/Electrical/Electrical Elements/Electrical Reference
  OP4 : ee_lib/Integrated Circuits/Band-Limited Op-Amp  A=1.8E6  Rin=4e6 Ohm  Rout=70 Ohm  Vmin=-24 V  Vmax=24 V  Vdotmax=2.8E6 V/s  f=8E6 Hz  V0=9.81 V
  Potentiometer : ee_lib/Passive/Potentiometer  nPorts=ee.enum.passive.potentiometer.nPorts.Three  R0=10E3 Ohm  Rw=1 Ohm  xmin=0  xmax=1  minResistance=1 Ohm  maxResistance=999 Ohm  xmin2port=0  xmax2port=1  Taper=ee.enum.passive.potentiometer.linOrLog.lin  Rcenter=200 Ohm  Gradient=ee.enum.passive.potentiometer.gradient.higherR
      settings: InternalSimscapePortConfiguration="{\"Bottom\":[],\"Left\":[{\"id\":\"pinL\",\"label\":\"L\",\"type\":\"foundation.electrical.electrical\"},{\"id\":\"W\",\"label\":\"W\",\"type\":\"foundation.electrical.electrical\"}],\"Right\":[{\"id\":\"pinR\",\"label\":\"R\",\"type\":\"foundation.electrical.electrical\"},{\"id\":\"x\",\"label\":\"x\",\"type\":\"input\"}],\"Top\":[]}"
  Simulink-PS Converter : nesl_utility/Simulink-PS Converter  PhysicalDomain=network_engine_domain  SubClassName=ps_input  LeftPortType=input  RightPortType=output  PseudoPeriodic=off  Frequencies=[]  NoiseDistribution=none  NoiseParameters=[]  Unit=1  AffineConversion=off  FilteringAndDerivatives=provide  SimscapeFilterOrder=1  InputFilterTimeConstant=0.001  UdotUserProvided=0
  g : PMIOPort  Side=Right
  in : PMIOPort  Port=2  Side=Left
  wires:
  input0/1 -> Simulink-PS Converter/1
  connections:
  Simulink-PS Converter/RConn1 -- Potentiometer/RConn2
  Potentiometer/LConn2 -- OP4/LConn1
  Electrical Reference4/LConn1 -- Potentiometer/LConn1
  OP4/RConn1 -- g/RConn1 -- OP4/LConn2
  in/RConn1 -- Potentiometer/RConn1

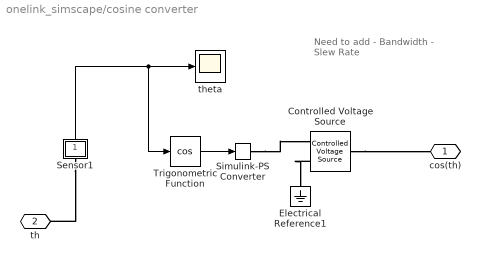
== system onelink_simscape/cosine converter ==
  note: Need to add
      | - Bandwidth
      | - Slew Rate
  Controlled Voltage Source : fl_lib/Electrical/Electrical Sources/Controlled Voltage Source
  Electrical Reference1 : fl_lib/Electrical/Electrical Elements/Electrical Reference
  Sensor1 : Subsystem
      mask Display: disp('S')
  Simulink-PS Converter : nesl_utility/Simulink-PS Converter  PhysicalDomain=network_engine_domain  SubClassName=ps_input  LeftPortType=input  RightPortType=output  PseudoPeriodic=off  Frequencies=[]  NoiseDistribution=none  NoiseParameters=[]  Unit=1  AffineConversion=off  FilteringAndDerivatives=provide  SimscapeFilterOrder=1  InputFilterTimeConstant=0.001  UdotUserProvided=0
  Trigonometric Function : Trigonometry  Operator=cos
  theta : Scope
      settings: ActiveDisplayYMinimum=-0.15074  ActiveDisplayYMaximum=0.77598  DataLoggingVariableName=ScopeData2
  cos(th) : PMIOPort  Side=Right
  th : PMIOPort  Port=2  Side=Left
  wires:
  Sensor1/1(Out1) -> Trigonometric Function/1, theta/1
  Trigonometric Function/1 -> Simulink-PS Converter/1
  connections:
  Controlled Voltage Source/RConn2 -- Electrical Reference1/LConn1
  Simulink-PS Converter/RConn1 -- Controlled Voltage Source/RConn1
  Sensor1/LConn1 -- th/RConn1
  Controlled Voltage Source/LConn1 -- cos(th)/RConn1

== system onelink_simscape/gain= -0.5（1） ==
  Electrical Reference1 : fl_lib/Electrical/Electrical Elements/Electrical Reference
  OP27 : ee_lib/Integrated Circuits/Band-Limited Op-Amp  A=1.8E6  Rin=4e6 Ohm  Rout=70 Ohm  Vmin=-24 V  Vmax=24 V  Vdotmax=2.8E6 V/s  f=8E6 Hz  V0=0 V
  s1 : fl_lib/Electrical/Electrical Elements/Resistor  R=1E3 Ohm  i_specify=off  i_priority=None  i=0 A  i_nominal_specify=off  i_nominal_value=1  i_nominal_unit=A  v_specify=off  v_priority=None  v=0 V  v_nominal_specify=off  v_nominal_value=1  v_nominal_unit=V
  s6 : fl_lib/Electrical/Electrical Elements/Resistor  R=0.5*1E3 Ohm  i_specify=off  i_priority=None  i=0 A  i_nominal_specify=off  i_nominal_value=1  i_nominal_unit=A  v_specify=off  v_priority=None  v=0 V  v_nominal_specify=off  v_nominal_value=1  v_nominal_unit=V
  out : PMIOPort  Side=Right
  in : PMIOPort  Port=2  Side=Left
  connections:
  OP27/LConn2 -- s1/RConn1 -- s6/LConn1
  s1/LConn1 -- in/RConn1
  Electrical Reference1/LConn1 -- OP27/LConn1
  out/RConn1 -- s6/RConn1 -- OP27/RConn1

== system onelink_simscape/gain= -0.5（2） ==
  Electrical Reference1 : fl_lib/Electrical/Electrical Elements/Electrical Reference
  OP27 : ee_lib/Integrated Circuits/Band-Limited Op-Amp  A=1.8E6  Rin=4e6 Ohm  Rout=70 Ohm  Vmin=-24 V  Vmax=24 V  Vdotmax=2.8E6 V/s  f=8E6 Hz  V0=0 V
  s1 : fl_lib/Electrical/Electrical Elements/Resistor  R=1E3 Ohm  i_specify=off  i_priority=None  i=0 A  i_nominal_specify=off  i_nominal_value=1  i_nominal_unit=A  v_specify=off  v_priority=None  v=0 V  v_nominal_specify=off  v_nominal_value=1  v_nominal_unit=V
  s6 : fl_lib/Electrical/Electrical Elements/Resistor  R=1*0.5E3 Ohm  i_specify=off  i_priority=None  i=0 A  i_nominal_specify=off  i_nominal_value=1  i_nominal_unit=A  v_specify=off  v_priority=None  v=0 V  v_nominal_specify=off  v_nominal_value=1  v_nominal_unit=V
  out : PMIOPort  Side=Right
  in : PMIOPort  Port=2  Side=Left
  connections:
  OP27/LConn2 -- s1/RConn1 -- s6/LConn1
  s1/LConn1 -- in/RConn1
  Electrical Reference1/LConn1 -- OP27/LConn1
  out/RConn1 -- s6/RConn1 -- OP27/RConn1

== system onelink_simscape/gain= -1//12（1） ==
  Electrical Reference1 : fl_lib/Electrical/Electrical Elements/Electrical Reference
  OP27 : ee_lib/Integrated Circuits/Band-Limited Op-Amp  A=1.8E6  Rin=4e6 Ohm  Rout=70 Ohm  Vmin=-24 V  Vmax=24 V  Vdotmax=2.8E6 V/s  f=8E6 Hz  V0=0 V
  s1 : fl_lib/Electrical/Electrical Elements/Resistor  R=1E3 Ohm  i_specify=off  i_priority=None  i=0 A  i_nominal_specify=off  i_nominal_value=1  i_nominal_unit=A  v_specify=off  v_priority=None  v=0 V  v_nominal_specify=off  v_nominal_value=1  v_nominal_unit=V
  s6 : fl_lib/Electrical/Electrical Elements/Resistor  R=1/12*1E3 Ohm  i_specify=off  i_priority=None  i=0 A  i_nominal_specify=off  i_nominal_value=1  i_nominal_unit=A  v_specify=off  v_priority=None  v=0 V  v_nominal_specify=off  v_nominal_value=1  v_nominal_unit=V
  out : PMIOPort  Side=Right
  in : PMIOPort  Port=2  Side=Left
  connections:
  OP27/LConn2 -- s1/RConn1 -- s6/LConn1
  s1/LConn1 -- in/RConn1
  Electrical Reference1/LConn1 -- OP27/LConn1
  out/RConn1 -- s6/RConn1 -- OP27/RConn1

== system onelink_simscape/gain= -1//12（2） ==
  Electrical Reference1 : fl_lib/Electrical/Electrical Elements/Electrical Reference
  OP27 : ee_lib/Integrated Circuits/Band-Limited Op-Amp  A=1.8E6  Rin=4e6 Ohm  Rout=70 Ohm  Vmin=-24 V  Vmax=24 V  Vdotmax=2.8E6 V/s  f=8E6 Hz  V0=0 V
  s1 : fl_lib/Electrical/Electrical Elements/Resistor  R=1E3 Ohm  i_specify=off  i_priority=None  i=0 A  i_nominal_specify=off  i_nominal_value=1  i_nominal_unit=A  v_specify=off  v_priority=None  v=0 V  v_nominal_specify=off  v_nominal_value=1  v_nominal_unit=V
  s6 : fl_lib/Electrical/Electrical Elements/Resistor  R=1/12*1E3 Ohm  i_specify=off  i_priority=None  i=0 A  i_nominal_specify=off  i_nominal_value=1  i_nominal_unit=A  v_specify=off  v_priority=None  v=0 V  v_nominal_specify=off  v_nominal_value=1  v_nominal_unit=V
  out : PMIOPort  Side=Right
  in : PMIOPort  Port=2  Side=Left
  connections:
  OP27/LConn2 -- s1/RConn1 -- s6/LConn1
  s1/LConn1 -- in/RConn1
  Electrical Reference1/LConn1 -- OP27/LConn1
  out/RConn1 -- s6/RConn1 -- OP27/RConn1

== system onelink_simscape/inverter1 ==
  Electrical Reference1 : fl_lib/Electrical/Electrical Elements/Electrical Reference
  OP2 : ee_lib/Integrated Circuits/Band-Limited Op-Amp  A=1.8E6  Rin=4e6 Ohm  Rout=70 Ohm  Vmin=-24 V  Vmax=24 V  Vdotmax=2.8E6 V/s  f=8E6 Hz  V0=0 V
  m1 : fl_lib/Electrical/Electrical Elements/Resistor  R=1E3 Ohm  i_specify=off  i_priority=None  i=0 A  i_nominal_specify=off  i_nominal_value=1  i_nominal_unit=A  v_specify=off  v_priority=None  v=0 V  v_nominal_specify=off  v_nominal_value=1  v_nominal_unit=V
  m2 : fl_lib/Electrical/Electrical Elements/Resistor  R=1E3 Ohm  i_specify=off  i_priority=None  i=0 A  i_nominal_specify=off  i_nominal_value=1  i_nominal_unit=A  v_specify=off  v_priority=None  v=0 V  v_nominal_specify=off  v_nominal_value=1  v_nominal_unit=V
  in : PMIOPort  Side=Left
  out : PMIOPort  Port=2  Side=Right
  connections:
  m1/LConn1 -- in/RConn1
  out/RConn1 -- OP2/RConn1 -- m2/LConn1
  OP2/LConn2 -- m1/RConn1 -- m2/RConn1
  OP2/LConn1 -- Electrical Reference1/LConn1

== system onelink_simscape/inverter10 ==
  Electrical Reference1 : fl_lib/Electrical/Electrical Elements/Electrical Reference
  OP2 : ee_lib/Integrated Circuits/Band-Limited Op-Amp  A=1.8E6  Rin=4e6 Ohm  Rout=70 Ohm  Vmin=-24 V  Vmax=24 V  Vdotmax=2.8E6 V/s  f=8E6 Hz  V0=0 V
  m1 : fl_lib/Electrical/Electrical Elements/Resistor  R=1E3 Ohm  i_specify=off  i_priority=None  i=0 A  i_nominal_specify=off  i_nominal_value=1  i_nominal_unit=A  v_specify=off  v_priority=None  v=0 V  v_nominal_specify=off  v_nominal_value=1  v_nominal_unit=V
  m2 : fl_lib/Electrical/Electrical Elements/Resistor  R=1E3 Ohm  i_specify=off  i_priority=None  i=0 A  i_nominal_specify=off  i_nominal_value=1  i_nominal_unit=A  v_specify=off  v_priority=None  v=0 V  v_nominal_specify=off  v_nominal_value=1  v_nominal_unit=V
  in : PMIOPort  Side=Left
  out : PMIOPort  Port=2  Side=Right
  connections:
  m1/LConn1 -- in/RConn1
  out/RConn1 -- OP2/RConn1 -- m2/LConn1
  OP2/LConn2 -- m1/RConn1 -- m2/RConn1
  OP2/LConn1 -- Electrical Reference1/LConn1

== system onelink_simscape/inverter11 ==
  Electrical Reference1 : fl_lib/Electrical/Electrical Elements/Electrical Reference
  OP2 : ee_lib/Integrated Circuits/Band-Limited Op-Amp  A=1.8E6  Rin=4e6 Ohm  Rout=70 Ohm  Vmin=-24 V  Vmax=24 V  Vdotmax=2.8E6 V/s  f=8E6 Hz  V0=0 V
  m1 : fl_lib/Electrical/Electrical Elements/Resistor  R=1E3 Ohm  i_specify=off  i_priority=None  i=0 A  i_nominal_specify=off  i_nominal_value=1  i_nominal_unit=A  v_specify=off  v_priority=None  v=0 V  v_nominal_specify=off  v_nominal_value=1  v_nominal_unit=V
  m2 : fl_lib/Electrical/Electrical Elements/Resistor  R=1E3 Ohm  i_specify=off  i_priority=None  i=0 A  i_nominal_specify=off  i_nominal_value=1  i_nominal_unit=A  v_specify=off  v_priority=None  v=0 V  v_nominal_specify=off  v_nominal_value=1  v_nominal_unit=V
  in : PMIOPort  Side=Left
  out : PMIOPort  Port=2  Side=Right
  connections:
  m1/LConn1 -- in/RConn1
  out/RConn1 -- OP2/RConn1 -- m2/LConn1
  OP2/LConn2 -- m1/RConn1 -- m2/RConn1
  OP2/LConn1 -- Electrical Reference1/LConn1

== system onelink_simscape/inverter12 ==
  Electrical Reference1 : fl_lib/Electrical/Electrical Elements/Electrical Reference
  OP2 : ee_lib/Integrated Circuits/Band-Limited Op-Amp  A=1.8E6  Rin=4e6 Ohm  Rout=70 Ohm  Vmin=-24 V  Vmax=24 V  Vdotmax=2.8E6 V/s  f=8E6 Hz  V0=0 V
  m1 : fl_lib/Electrical/Electrical Elements/Resistor  R=1E3 Ohm  i_specify=off  i_priority=None  i=0 A  i_nominal_specify=off  i_nominal_value=1  i_nominal_unit=A  v_specify=off  v_priority=None  v=0 V  v_nominal_specify=off  v_nominal_value=1  v_nominal_unit=V
  m2 : fl_lib/Electrical/Electrical Elements/Resistor  R=1E3 Ohm  i_specify=off  i_priority=None  i=0 A  i_nominal_specify=off  i_nominal_value=1  i_nominal_unit=A  v_specify=off  v_priority=None  v=0 V  v_nominal_specify=off  v_nominal_value=1  v_nominal_unit=V
  in : PMIOPort  Side=Left
  out : PMIOPort  Port=2  Side=Right
  connections:
  m1/LConn1 -- in/RConn1
  out/RConn1 -- OP2/RConn1 -- m2/LConn1
  OP2/LConn2 -- m1/RConn1 -- m2/RConn1
  OP2/LConn1 -- Electrical Reference1/LConn1

== system onelink_simscape/inverter13 ==
  Electrical Reference1 : fl_lib/Electrical/Electrical Elements/Electrical Reference
  OP2 : ee_lib/Integrated Circuits/Band-Limited Op-Amp  A=1.8E6  Rin=4e6 Ohm  Rout=70 Ohm  Vmin=-24 V  Vmax=24 V  Vdotmax=2.8E6 V/s  f=8E6 Hz  V0=0 V
  m1 : fl_lib/Electrical/Electrical Elements/Resistor  R=1E3 Ohm  i_specify=off  i_priority=None  i=0 A  i_nominal_specify=off  i_nominal_value=1  i_nominal_unit=A  v_specify=off  v_priority=None  v=0 V  v_nominal_specify=off  v_nominal_value=1  v_nominal_unit=V
  m2 : fl_lib/Electrical/Electrical Elements/Resistor  R=1E3 Ohm  i_specify=off  i_priority=None  i=0 A  i_nominal_specify=off  i_nominal_value=1  i_nominal_unit=A  v_specify=off  v_priority=None  v=0 V  v_nominal_specify=off  v_nominal_value=1  v_nominal_unit=V
  in : PMIOPort  Side=Left
  out : PMIOPort  Port=2  Side=Right
  connections:
  m1/LConn1 -- in/RConn1
  out/RConn1 -- OP2/RConn1 -- m2/LConn1
  OP2/LConn2 -- m1/RConn1 -- m2/RConn1
  OP2/LConn1 -- Electrical Reference1/LConn1

== system onelink_simscape/inverter14 ==
  Electrical Reference1 : fl_lib/Electrical/Electrical Elements/Electrical Reference
  OP2 : ee_lib/Integrated Circuits/Band-Limited Op-Amp  A=1.8E6  Rin=4e6 Ohm  Rout=70 Ohm  Vmin=-24 V  Vmax=24 V  Vdotmax=2.8E6 V/s  f=8E6 Hz  V0=0 V
  m1 : fl_lib/Electrical/Electrical Elements/Resistor  R=1E3 Ohm  i_specify=off  i_priority=None  i=0 A  i_nominal_specify=off  i_nominal_value=1  i_nominal_unit=A  v_specify=off  v_priority=None  v=0 V  v_nominal_specify=off  v_nominal_value=1  v_nominal_unit=V
  m2 : fl_lib/Electrical/Electrical Elements/Resistor  R=1E3 Ohm  i_specify=off  i_priority=None  i=0 A  i_nominal_specify=off  i_nominal_value=1  i_nominal_unit=A  v_specify=off  v_priority=None  v=0 V  v_nominal_specify=off  v_nominal_value=1  v_nominal_unit=V
  in : PMIOPort  Side=Left
  out : PMIOPort  Port=2  Side=Right
  connections:
  m1/LConn1 -- in/RConn1
  out/RConn1 -- OP2/RConn1 -- m2/LConn1
  OP2/LConn2 -- m1/RConn1 -- m2/RConn1
  OP2/LConn1 -- Electrical Reference1/LConn1

== system onelink_simscape/inverter15 ==
  Electrical Reference1 : fl_lib/Electrical/Electrical Elements/Electrical Reference
  OP2 : ee_lib/Integrated Circuits/Band-Limited Op-Amp  A=1.8E6  Rin=4e6 Ohm  Rout=70 Ohm  Vmin=-24 V  Vmax=24 V  Vdotmax=2.8E6 V/s  f=8E6 Hz  V0=0 V
  m1 : fl_lib/Electrical/Electrical Elements/Resistor  R=1E3 Ohm  i_specify=off  i_priority=None  i=0 A  i_nominal_specify=off  i_nominal_value=1  i_nominal_unit=A  v_specify=off  v_priority=None  v=0 V  v_nominal_specify=off  v_nominal_value=1  v_nominal_unit=V
  m2 : fl_lib/Electrical/Electrical Elements/Resistor  R=1E3 Ohm  i_specify=off  i_priority=None  i=0 A  i_nominal_specify=off  i_nominal_value=1  i_nominal_unit=A  v_specify=off  v_priority=None  v=0 V  v_nominal_specify=off  v_nominal_value=1  v_nominal_unit=V
  in : PMIOPort  Side=Left
  out : PMIOPort  Port=2  Side=Right
  connections:
  m1/LConn1 -- in/RConn1
  out/RConn1 -- OP2/RConn1 -- m2/LConn1
  OP2/LConn2 -- m1/RConn1 -- m2/RConn1
  OP2/LConn1 -- Electrical Reference1/LConn1

== system onelink_simscape/inverter2 ==
  Electrical Reference1 : fl_lib/Electrical/Electrical Elements/Electrical Reference
  OP2 : ee_lib/Integrated Circuits/Band-Limited Op-Amp  A=1.8E6  Rin=4e6 Ohm  Rout=70 Ohm  Vmin=-24 V  Vmax=24 V  Vdotmax=2.8E6 V/s  f=8E6 Hz  V0=0 V
  m1 : fl_lib/Electrical/Electrical Elements/Resistor  R=1E3 Ohm  i_specify=off  i_priority=None  i=0 A  i_nominal_specify=off  i_nominal_value=1  i_nominal_unit=A  v_specify=off  v_priority=None  v=0 V  v_nominal_specify=off  v_nominal_value=1  v_nominal_unit=V
  m2 : fl_lib/Electrical/Electrical Elements/Resistor  R=1E3 Ohm  i_specify=off  i_priority=None  i=0 A  i_nominal_specify=off  i_nominal_value=1  i_nominal_unit=A  v_specify=off  v_priority=None  v=0 V  v_nominal_specify=off  v_nominal_value=1  v_nominal_unit=V
  in : PMIOPort  Side=Left
  out : PMIOPort  Port=2  Side=Right
  connections:
  m1/LConn1 -- in/RConn1
  out/RConn1 -- OP2/RConn1 -- m2/LConn1
  OP2/LConn2 -- m1/RConn1 -- m2/RConn1
  OP2/LConn1 -- Electrical Reference1/LConn1

== system onelink_simscape/inverter3 ==
  Electrical Reference1 : fl_lib/Electrical/Electrical Elements/Electrical Reference
  OP2 : ee_lib/Integrated Circuits/Band-Limited Op-Amp  A=1.8E6  Rin=4e6 Ohm  Rout=70 Ohm  Vmin=-24 V  Vmax=24 V  Vdotmax=2.8E6 V/s  f=8E6 Hz  V0=0 V
  m1 : fl_lib/Electrical/Electrical Elements/Resistor  R=1E3 Ohm  i_specify=off  i_priority=None  i=0 A  i_nominal_specify=off  i_nominal_value=1  i_nominal_unit=A  v_specify=off  v_priority=None  v=0 V  v_nominal_specify=off  v_nominal_value=1  v_nominal_unit=V
  m2 : fl_lib/Electrical/Electrical Elements/Resistor  R=1E3 Ohm  i_specify=off  i_priority=None  i=0 A  i_nominal_specify=off  i_nominal_value=1  i_nominal_unit=A  v_specify=off  v_priority=None  v=0 V  v_nominal_specify=off  v_nominal_value=1  v_nominal_unit=V
  in : PMIOPort  Side=Left
  out : PMIOPort  Port=2  Side=Right
  connections:
  m1/LConn1 -- in/RConn1
  out/RConn1 -- OP2/RConn1 -- m2/LConn1
  OP2/LConn2 -- m1/RConn1 -- m2/RConn1
  OP2/LConn1 -- Electrical Reference1/LConn1

== system onelink_simscape/inverter4 ==
  Electrical Reference1 : fl_lib/Electrical/Electrical Elements/Electrical Reference
  OP2 : ee_lib/Integrated Circuits/Band-Limited Op-Amp  A=1.8E6  Rin=4e6 Ohm  Rout=70 Ohm  Vmin=-24 V  Vmax=24 V  Vdotmax=2.8E6 V/s  f=8E6 Hz  V0=0 V
  m1 : fl_lib/Electrical/Electrical Elements/Resistor  R=1E3 Ohm  i_specify=off  i_priority=None  i=0 A  i_nominal_specify=off  i_nominal_value=1  i_nominal_unit=A  v_specify=off  v_priority=None  v=0 V  v_nominal_specify=off  v_nominal_value=1  v_nominal_unit=V
  m2 : fl_lib/Electrical/Electrical Elements/Resistor  R=1E3 Ohm  i_specify=off  i_priority=None  i=0 A  i_nominal_specify=off  i_nominal_value=1  i_nominal_unit=A  v_specify=off  v_priority=None  v=0 V  v_nominal_specify=off  v_nominal_value=1  v_nominal_unit=V
  in : PMIOPort  Side=Left
  out : PMIOPort  Port=2  Side=Right
  connections:
  m1/LConn1 -- in/RConn1
  out/RConn1 -- OP2/RConn1 -- m2/LConn1
  OP2/LConn2 -- m1/RConn1 -- m2/RConn1
  OP2/LConn1 -- Electrical Reference1/LConn1
